simulink model "Version_final_sous_modele"  (R2018b)
settings: Solver=VariableStepAuto  StartTime=0.0  StopTime=10.0  RelTol=1e-3
values from neighbouring files (symbols this model uses):
  fa_clu_pos = [1 1 0.7 0.5 0.3 0 0]    [AxelSplitHEVv4_NEDC_18_06_15.mat]
  fa_clu_pv = [0 0.1 0.3 0.5 0.7 0.9 1]    [AxelSplitHEVv4_NEDC_18_06_15.mat]
  fa_differential_ratio = FDR.fa_differential_ratio    [Algorithme_eff.m]    (also in AxelSplitHEVv4_NEDC_18_06_15.mat = 3.72; fa_differential_ratio.mat = 3.72)
  fa_gearbox_efficiency = 0.92    [AxelSplitHEVv4_NEDC_18_06_15.mat]
  fa_gearbox_ratio = FGR.fa_gearbox_ratio    [Algorithme_eff.m]    (also in AxelSplitHEVv4_NEDC_18_06_15.mat = [0 3.98 2.21 1.47 1.1 0.89 0.75]; fa_gearbox_ratio.mat = [0 3.98 2.21 1.47 1.1 0.89 0.75])
  fa_ice_inertia = 0.058    [AxelSplitHEVv4_NEDC_18_06_15.mat]
  fa_max_tq_clu = 206    [AxelSplitHEVv4_NEDC_18_06_15.mat]
  fa_tau_ice = 0.0333    [AxelSplitHEVv4_NEDC_18_06_15.mat]
  hev_dt = 0.01    [AxelSplitHEVv4_NEDC_18_06_15.mat]
  pla_csat = 1.2    [AxelSplitHEVv4_NEDC_18_06_15.mat]
  pla_equivalent_weight = 1250    [AxelSplitHEVv4_NEDC_18_06_15.mat]
  pla_f = 0.0035272    [AxelSplitHEVv4_NEDC_18_06_15.mat]
  pla_k = 0.0002318    [AxelSplitHEVv4_NEDC_18_06_15.mat]
  pla_kaero = 0.52992    [AxelSplitHEVv4_NEDC_18_06_15.mat]
  pla_max_f_brakes = 1000    [AxelSplitHEVv4_NEDC_18_06_15.mat]
  pla_wheel_radius = 0.314    [AxelSplitHEVv4_NEDC_18_06_15.mat]
  ra_differential_ratio = RDR.ra_differential_ratio    [Algorithme_eff.m]    (also in AxelSplitHEVv4_NEDC_18_06_15.mat = 10; ra_differential_ratio.mat = 10)
  ra_electrical_machine_tau = 0.1    [AxelSplitHEVv4_NEDC_18_06_15.mat]
  ra_transmission_efficiency = 0.92    [AxelSplitHEVv4_NEDC_18_06_15.mat]
undefined symbols (not defined in the file or in its folder): DiscIntNeverNeededParam
libraries: simulink x4
settings Model: Creator=smouline  LastModifiedBy=test
settings SFSimCC: SimUseLocalCustomCode=off
settings RTWCC: RTWUseLocalCustomCode=off
settings CodeAppCC: StateflowObjectComments=on

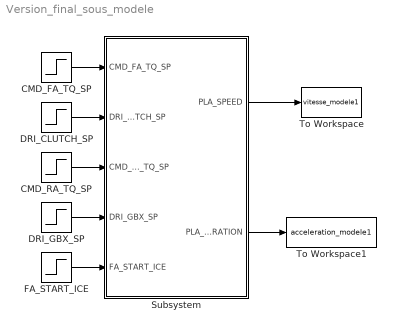
== system Version_final_sous_modele ==
  CMD_FA_TQ_SP : Step  Time=50.1  After=5  SampleTime=0
  CMD_RA_TQ_SP : Step  Time=2  After=10  SampleTime=0
  DRI_CLUTCH_SP : Step  Time=50  Before=1  SampleTime=0
  DRI_GBX_SP : Step  Time=50  Before=1  SampleTime=0
  FA_START_ICE : Step  Time=50  SampleTime=0
  Subsystem : Subsystem
  To Workspace : ToWorkspace  VariableName=vitesse_modele1  SampleTime=-1
  To Workspace1 : ToWorkspace  VariableName=acceleration_modele1  SampleTime=-1
  wires:
  Subsystem/1(PLA_SPEED) -> To Workspace/1
  DRI_GBX_SP/1 -> Subsystem/4(DRI_GBX_SP)
  DRI_CLUTCH_SP/1 -> Subsystem/2(DRI_CLUTCH_SP)
  CMD_FA_TQ_SP/1 -> Subsystem/1(CMD_FA_TQ_SP)
  CMD_RA_TQ_SP/1 -> Subsystem/3(CMD_RA_TQ_SP)
  Subsystem/2(PLA_ACCELERATION) -> To Workspace1/1
  FA_START_ICE/1 -> Subsystem/5(FA_START_ICE)

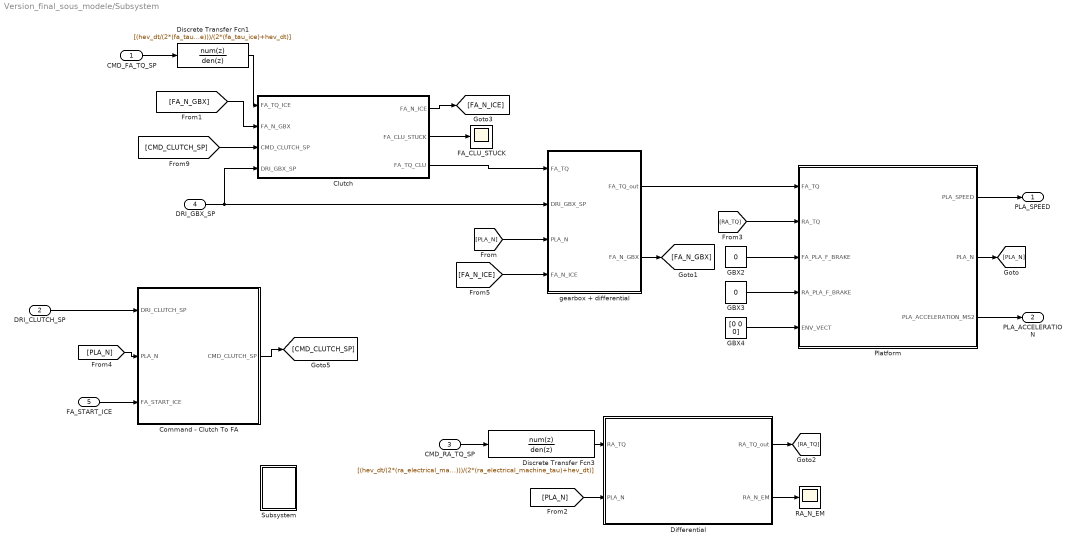
== system Version_final_sous_modele/Subsystem ==
  CMD_FA_TQ_SP : Inport
  DRI_CLUTCH_SP : Inport  Port=2
  CMD_RA_TQ_SP : Inport  Port=3
  DRI_GBX_SP : Inport  Port=4
  FA_START_ICE : Inport  Port=5
  Clutch : Subsystem
  Command - Clutch To FA : Subsystem
  Differential : Subsystem
  Discrete Transfer Fcn1 : DiscreteTransferFcn  Numerator=[(hev_dt/(2*(fa_tau_ice)+hev_dt)) (hev_dt/(2*(fa_tau_ice)+hev_dt))]  Denominator=[1 ((hev_dt-2*(fa_tau_ice)))/(2*(fa_tau_ice)+hev_dt)]  SampleTime=hev_dt
  Discrete Transfer Fcn3 : DiscreteTransferFcn  Numerator=[(hev_dt/(2*(ra_electrical_machine_tau)+hev_dt)) (hev_dt/(2*(ra_electrical_machine_tau)+hev_dt))]  Denominator=[1 ((hev_dt-2*(ra_electrical_machine_tau)))/(2*(ra_electrical_machine_tau)+hev_dt)]  SampleTime=hev_dt
  FA_CLU_STUCK : Scope
  GBX2 : Constant  Value=0
  GBX3 : Constant  Value=0
  GBX4 : Constant  Value=[0 0 0]
  Platform : Subsystem
  RA_N_EM : Scope
  Subsystem : Subsystem
      settings: OpenFcn=open('Documents/Subsystem (extraction of the useful blocs for the clutch’s command).pdf')
      mask Display: fprintf('DOC')
  gearbox + differential : Subsystem
  PLA_SPEED : Outport
  PLA_ACCELERATION : Outport  Port=2
  wires:
  DRI_GBX_SP/1 -> gearbox + differential/2(DRI_GBX_SP), Clutch/4(DRI_GBX_SP)
  Command - Clutch To FA/1("CMD_CLUTCH_SP ") -> [CMD_CLUTCH_SP]
  GBX2/1 -> Platform/3(FA_PLA_F_BRAKE)
  [RA_TQ] -> Platform/2(RA_TQ)
  Differential/2(RA_N_EM) -> RA_N_EM/1
  Platform/3(PLA_ACCELERATION_MS2) -> PLA_ACCELERATION/1
  Differential/1(RA_TQ_out) -> [RA_TQ]
  GBX4/1 -> Platform/5(ENV_VECT)
  gearbox + differential/1("FA_TQ_out ") -> Platform/1(FA_TQ)
  gearbox + differential/2(FA_N_GBX) -> [FA_N_GBX]
  Platform/1(PLA_SPEED) -> PLA_SPEED/1
  [PLA_N] -> gearbox + differential/3(PLA_N)
  [PLA_N] -> Command - Clutch To FA/2(PLA_N)
  Platform/2(PLA_N) -> [PLA_N]
  [FA_N_GBX] -> Clutch/2(FA_N_GBX)
  Discrete Transfer Fcn3/1 -> Differential/1(RA_TQ)
  [FA_N_ICE] -> gearbox + differential/4(FA_N_ICE)
  [PLA_N] -> Differential/2(PLA_N)
  Discrete Transfer Fcn1/1 -> Clutch/1(FA_TQ_ICE)
  Clutch/1(FA_N_ICE) -> [FA_N_ICE]
  CMD_FA_TQ_SP/1 -> Discrete Transfer Fcn1/1
  Clutch/3(FA_TQ_CLU) -> gearbox + differential/1(FA_TQ)
  GBX3/1 -> Platform/4(RA_PLA_F_BRAKE)
  CMD_RA_TQ_SP/1 -> Discrete Transfer Fcn3/1
  [CMD_CLUTCH_SP] -> Clutch/3(CMD_CLUTCH_SP)
  Clutch/2(FA_CLU_STUCK) -> FA_CLU_STUCK/1
  DRI_CLUTCH_SP/1 -> Command - Clutch To FA/1(DRI_CLUTCH_SP)
  FA_START_ICE/1 -> Command - Clutch To FA/3(FA_START_ICE)

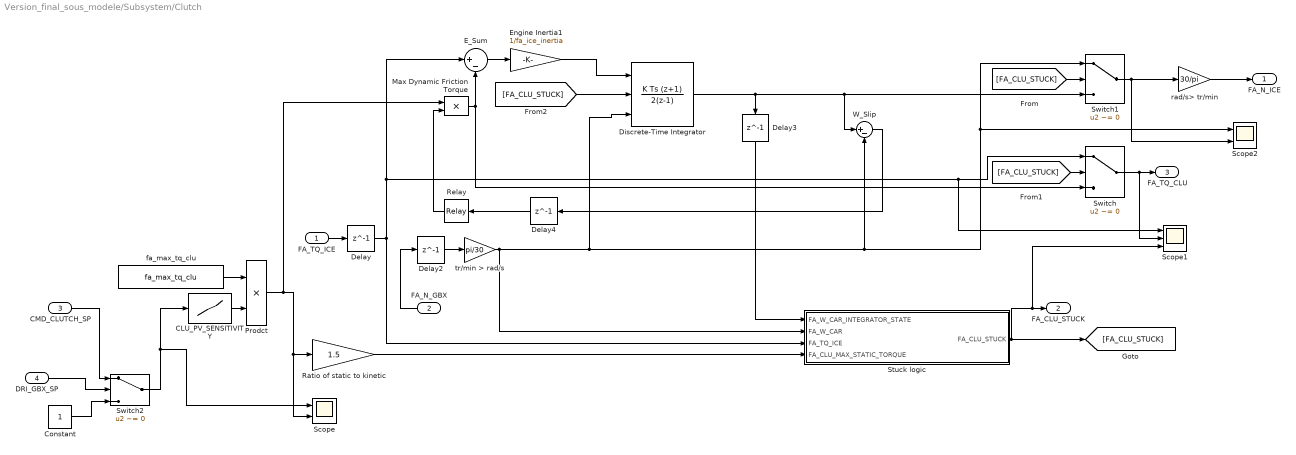
== system Version_final_sous_modele/Subsystem/Clutch ==
  FA_TQ_ICE : Inport
  FA_N_GBX : Inport  Port=2
  CMD_CLUTCH_SP : Inport  Port=3
  DRI_GBX_SP : Inport  Port=4
  " tr/min > rad/s" : Gain  Gain=pi/30  SampleTime=hev_dt
  CLU_PV_SENSITIVITY : Lookup_n-D  NumberOfTableDimensions=1  BreakpointsForDimension1=fa_clu_pv  Table=fa_clu_pos  ExtrapMethod=Clip  UseLastTableValue=on  SampleTime=hev_dt  RndMeth=Simplest  InputSameDT=on
  Constant : Constant
  Delay{,2..4} (4 alike) : Delay  DelayLength=1  SampleTime=hev_dt
  Discrete-Time Integrator : DiscreteIntegrator  IntegratorMethod=Integration: Trapezoidal  ExternalReset=falling  InitialConditionSource=external  SampleTime=hev_dt  ICPrevOutput=DiscIntNeverNeededParam  ICPrevScaledInput=DiscIntNeverNeededParam
  E_Sum : Sum  Inputs=|+-  SampleTime=hev_dt  SaturateOnIntegerOverflow=on  InputSameDT=on  OutDataTypeStr=Inherit: Same as first input
  Engine Inertia1 : Gain  Gain=1/fa_ice_inertia  SampleTime=hev_dt  SaturateOnIntegerOverflow=on  OutDataTypeStr=Inherit: Same as input  ParamDataTypeStr=Inherit: Same as input
  Max Dynamic Friction Torque : Product  SampleTime=hev_dt  SaturateOnIntegerOverflow=on  RndMeth=Zero  InputSameDT=on  OutDataTypeStr=Inherit: Same as first input
  Prodct : Product  SampleTime=hev_dt  RndMeth=Zero
  Ratio of static to kinetic : Gain  Gain=1.5  SampleTime=hev_dt  SaturateOnIntegerOverflow=on  OutDataTypeStr=Inherit: Same as input  ParamDataTypeStr=Inherit: Same as input
  Relay : Relay  OnSwitchValue=0  OffSwitchValue=0  OffOutputValue=-1  SampleTime=hev_dt
  Scope : Scope  NumInputPorts=2
  Scope1 : Scope  NumInputPorts=3
  Scope2 : Scope  NumInputPorts=2
  Stuck logic : Subsystem
  Switch : Switch  Criteria=u2 ~= 0  SampleTime=hev_dt
  Switch1 : Switch  Criteria=u2 ~= 0  SampleTime=hev_dt
  Switch2 : Switch  Criteria=u2 ~= 0
  W_Slip : Sum  Inputs=|+-  SampleTime=hev_dt  SaturateOnIntegerOverflow=on  InputSameDT=on  OutDataTypeStr=Inherit: Same as first input
  fa_max_tq_clu : Constant  Value=fa_max_tq_clu
  rad/s> tr/min : Gain  Gain=30/pi  SampleTime=hev_dt
  FA_N_ICE : Outport
  FA_CLU_STUCK : Outport  Port=2
  FA_TQ_CLU : Outport  Port=3
  wires:
  FA_TQ_ICE/1 -> Delay/1
  Switch1/1 -> Scope2/2, rad/s> tr/min/1
  Switch/1 -> Scope1/2, FA_TQ_CLU/1
  fa_max_tq_clu/1 -> Prodct/1
  Prodct/1 -> Max Dynamic Friction Torque/1, Scope/2, Ratio of static to kinetic/1
  Delay/1 -> E_Sum/1, Scope1/1, Switch/1, Stuck logic/3(FA_TQ_ICE)
  " tr/min > rad/s"/1 -> Discrete-Time Integrator/3, Switch1/1, Scope2/1, W_Slip/2, Stuck logic/2(FA_W_CAR)
  rad/s> tr/min/1 -> FA_N_ICE/1
  Ratio of static to kinetic/1 -> Stuck logic/4(FA_CLU_MAX_STATIC_TORQUE)
  E_Sum/1 -> Engine Inertia1/1
  Engine Inertia1/1 -> Discrete-Time Integrator/1
  Relay/1 -> Max Dynamic Friction Torque/2
  Max Dynamic Friction Torque/1 -> E_Sum/2, Switch/3
  [FA_CLU_STUCK] -> Switch1/2
  [FA_CLU_STUCK] -> Switch/2
  [FA_CLU_STUCK] -> Discrete-Time Integrator/2
  W_Slip/1 -> Delay4/1
  Delay2/1 -> " tr/min > rad/s"/1
  FA_N_GBX/1 -> Delay2/1
  CMD_CLUTCH_SP/1 -> Switch2/1
  Discrete-Time Integrator/1 -> W_Slip/1, Switch1/3, Delay3/1
  Delay3/1 -> Stuck logic/1(FA_W_CAR_INTEGRATOR_STATE)
  Switch2/1 -> Scope/1, CLU_PV_SENSITIVITY/1
  DRI_GBX_SP/1 -> Switch2/2
  Constant/1 -> Switch2/3
  Delay4/1 -> Relay/1
  CLU_PV_SENSITIVITY/1 -> Prodct/2
  Stuck logic/1(FA_CLU_STUCK) -> [FA_CLU_STUCK], Scope1/3, FA_CLU_STUCK/1

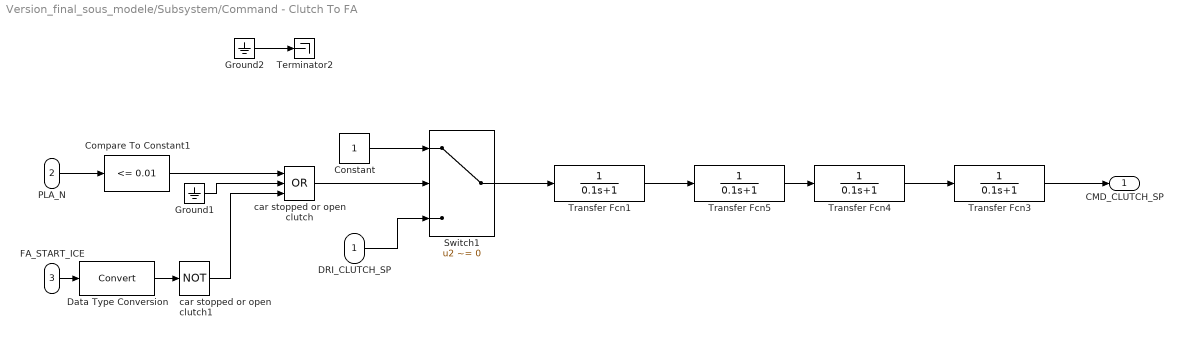
== system Version_final_sous_modele/Subsystem/Command - Clutch To FA ==
  DRI_CLUTCH_SP : Inport
  PLA_N : Inport  Port=2
  FA_START_ICE : Inport  Port=3
  Compare To Constant1 : simulink/Logic and Bit Operations/Compare To Constant  relop=<=  const=0.01  OutDataTypeStr=uint8
  Constant : Constant
  Data Type Conversion : DataTypeConversion
  Ground1 : Ground
  Ground2 : Ground
  Switch1 : Switch  Criteria=u2 ~= 0  Threshold=1
  Terminator2 : Terminator
  Transfer Fcn{1,3..5} (4 alike) : TransferFcn  Denominator=[0.1 1]
  car stopped or open clutch : Logic  Operator=OR  Inputs=3  AllPortsSameDT=off  OutDataTypeStr=boolean
  car stopped or open clutch1 : Logic  Operator=NOT  Inputs=3  AllPortsSameDT=off  OutDataTypeStr=boolean
  "CMD_CLUTCH_SP " : Outport
  wires:
  PLA_N/1 -> Compare To Constant1/1
  FA_START_ICE/1 -> Data Type Conversion/1
  Data Type Conversion/1 -> car stopped or open clutch1/1
  Compare To Constant1/1 -> car stopped or open clutch/1
  Ground1/1 -> car stopped or open clutch/2
  car stopped or open clutch1/1 -> car stopped or open clutch/3
  Ground2/1 -> Terminator2/1
  Constant/1 -> Switch1/1
  car stopped or open clutch/1 -> Switch1/2
  DRI_CLUTCH_SP/1 -> Switch1/3
  Transfer Fcn5/1 -> Transfer Fcn4/1
  Transfer Fcn4/1 -> Transfer Fcn3/1
  Transfer Fcn1/1 -> Transfer Fcn5/1
  Switch1/1 -> Transfer Fcn1/1
  Transfer Fcn3/1 -> "CMD_CLUTCH_SP "/1

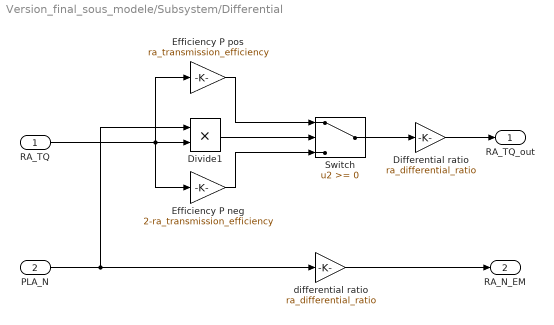
== system Version_final_sous_modele/Subsystem/Differential ==
  RA_TQ : Inport
  PLA_N : Inport  Port=2
  Differential ratio : Gain  Gain=ra_differential_ratio  SampleTime=hev_dt
  Divide1 : Product  SampleTime=hev_dt
  Efficiency P neg : Gain  Gain=2-ra_transmission_efficiency  SampleTime=hev_dt
  Efficiency P pos : Gain  Gain=ra_transmission_efficiency  SampleTime=hev_dt
  Switch : Switch  SampleTime=hev_dt
  differential ratio : Gain  Gain=ra_differential_ratio  SampleTime=hev_dt
  RA_TQ_out : Outport
  RA_N_EM : Outport  Port=2
  wires:
  RA_TQ/1 -> Divide1/2, Efficiency P neg/1, Efficiency P pos/1
  Efficiency P pos/1 -> Switch/1
  Efficiency P neg/1 -> Switch/3
  Divide1/1 -> Switch/2
  Switch/1 -> Differential ratio/1
  PLA_N/1 -> Divide1/1, differential ratio/1
  Differential ratio/1 -> RA_TQ_out/1
  differential ratio/1 -> RA_N_EM/1

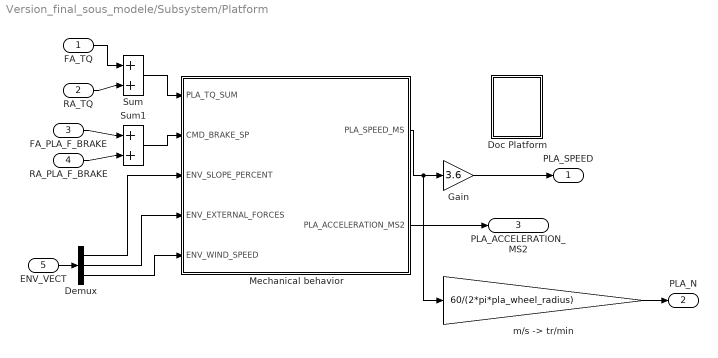
== system Version_final_sous_modele/Subsystem/Platform ==
  FA_TQ : Inport
  RA_TQ : Inport  Port=2
  FA_PLA_F_BRAKE : Inport  Port=3
  RA_PLA_F_BRAKE : Inport  Port=4
  ENV_VECT : Inport  Port=5
  Demux : Demux  Outputs=3
  Doc Platform : Subsystem
      settings: OpenFcn=open('Documents\Platform.pdf')
      mask Display: fprintf('DOC')
  Gain : Gain  Gain=3.6  SampleTime=hev_dt
  Mechanical behavior : Subsystem
  Sum : Sum  Inputs=+|+  SampleTime=hev_dt
  Sum1 : Sum  Inputs=+|+  SampleTime=hev_dt
  "m/s -> tr/min" : Gain  Gain=60/(2*pi*pla_wheel_radius)  SampleTime=hev_dt
  PLA_SPEED : Outport
  PLA_N : Outport  Port=2
  PLA_ACCELERATION_MS2 : Outport  Port=3
  wires:
  Mechanical behavior/1(PLA_SPEED_MS) -> Gain/1, "m/s -> tr/min"/1
  ENV_VECT/1 -> Demux/1
  Gain/1 -> PLA_SPEED/1
  "m/s -> tr/min"/1 -> PLA_N/1
  Sum/1 -> Mechanical behavior/1(PLA_TQ_SUM)
  RA_TQ/1 -> Sum/2
  FA_TQ/1 -> Sum/1
  Sum1/1 -> Mechanical behavior/2(CMD_BRAKE_SP)
  RA_PLA_F_BRAKE/1 -> Sum1/2
  FA_PLA_F_BRAKE/1 -> Sum1/1
  Mechanical behavior/2(PLA_ACCELERATION_MS2) -> PLA_ACCELERATION_MS2/1
  Demux/3 -> Mechanical behavior/5(ENV_WIND_SPEED)
  Demux/2 -> Mechanical behavior/4(ENV_EXTERNAL_FORCES)
  Demux/1 -> Mechanical behavior/3(ENV_SLOPE_PERCENT)

== system Version_final_sous_modele/Subsystem/Subsystem ==

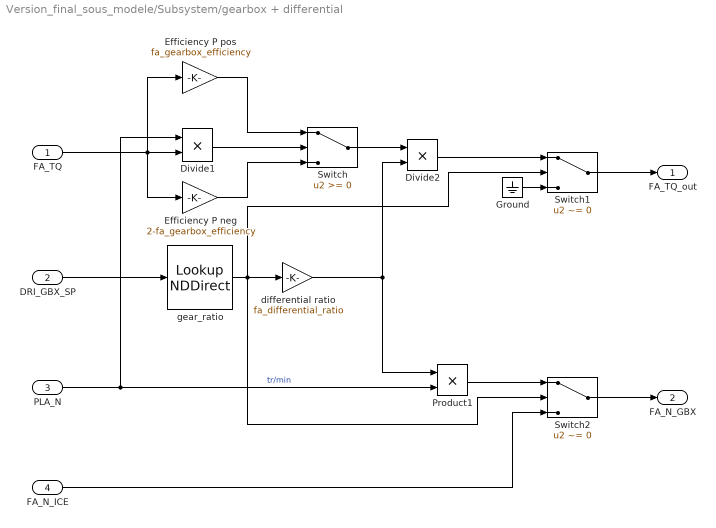
== system Version_final_sous_modele/Subsystem/gearbox + differential ==
  FA_TQ : Inport
  DRI_GBX_SP : Inport  Port=2
  PLA_N : Inport  Port=3
  FA_N_ICE : Inport  Port=4
  " gear_ratio" : LookupNDDirect  NumberOfTableDimensions=1  Table=fa_gearbox_ratio  SampleTime=hev_dt
  Divide1 : Product  SampleTime=hev_dt
  Divide2 : Product  Inputs=**  SampleTime=hev_dt
  Efficiency P neg : Gain  Gain=2-fa_gearbox_efficiency  SampleTime=hev_dt
  Efficiency P pos : Gain  Gain=fa_gearbox_efficiency  SampleTime=hev_dt
  Ground : Ground
  Product1 : Product  SampleTime=hev_dt  RndMeth=Zero
  Switch : Switch  SampleTime=hev_dt
  Switch1 : Switch  Criteria=u2 ~= 0  SampleTime=hev_dt
  Switch2 : Switch  Criteria=u2 ~= 0  SampleTime=hev_dt
  differential ratio : Gain  Gain=fa_differential_ratio  SampleTime=hev_dt
  "FA_TQ_out " : Outport
  FA_N_GBX : Outport  Port=2
  wires:
  DRI_GBX_SP/1 -> " gear_ratio"/1
  " gear_ratio"/1 -> Switch1/2, differential ratio/1, Switch2/2
  differential ratio/1 -> Divide2/2, Product1/1
  Divide2/1 -> Switch1/1
  FA_TQ/1 -> Divide1/2, Efficiency P neg/1, Efficiency P pos/1
  Efficiency P pos/1 -> Switch/1
  Efficiency P neg/1 -> Switch/3
  Divide1/1 -> Switch/2
  Switch/1 -> Divide2/1
  Product1/1 -> Switch2/1
  PLA_N/1 -> Product1/2, Divide1/1  "tr/min"
  Switch1/1 -> "FA_TQ_out "/1
  Ground/1 -> Switch1/3
  Switch2/1 -> FA_N_GBX/1
  FA_N_ICE/1 -> Switch2/3

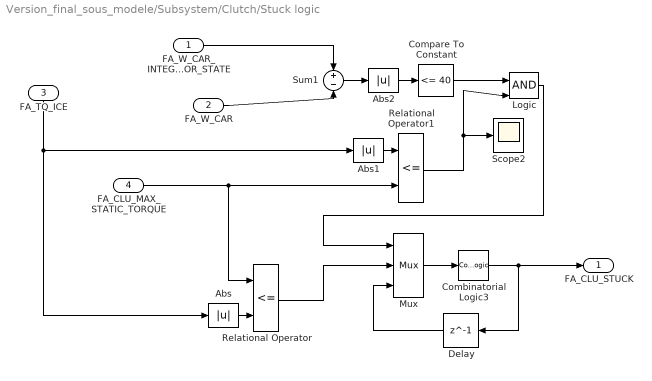
== system Version_final_sous_modele/Subsystem/Clutch/Stuck logic ==
  FA_W_CAR_INTEGRATOR_STATE : Inport
  FA_W_CAR : Inport  Port=2
  FA_TQ_ICE : Inport  Port=3
  FA_CLU_MAX_STATIC_TORQUE : Inport  Port=4
  Abs : Abs  SampleTime=hev_dt  SaturateOnIntegerOverflow=on
  Abs1 : Abs  SampleTime=hev_dt  SaturateOnIntegerOverflow=on
  Abs2 : Abs  SampleTime=hev_dt  SaturateOnIntegerOverflow=on
  Combinatorial Logic3 : CombinatorialLogic  Description=TRUTH_TABLE_FROM_FABIEN  TruthTable=[0;1;0;0;1;1;0;1]  SampleTime=hev_dt
  Compare To Constant : simulink/Logic and Bit Operations/Compare To Constant  relop=<=  const=40  OutDataTypeStr=boolean
  Delay : Delay  DelayLength=1  SampleTime=hev_dt
  Logic : Logic  IconShape=distinctive  SampleTime=hev_dt
  Mux : Mux  Inputs=3
  Relational Operator : RelationalOperator  Operator=<=  SampleTime=hev_dt  RndMeth=Nearest  InputSameDT=on
  Relational Operator1 : RelationalOperator  Operator=<=  SampleTime=hev_dt  RndMeth=Nearest  InputSameDT=on
  Scope2 : Scope
  Sum1 : Sum  Inputs=+-  SampleTime=hev_dt  SaturateOnIntegerOverflow=on  InputSameDT=on  OutDataTypeStr=Inherit: Same as first input
  FA_CLU_STUCK : Outport
  wires:
  FA_CLU_MAX_STATIC_TORQUE/1 -> Relational Operator1/2, Relational Operator/1
  Sum1/1 -> Abs2/1
  Abs1/1 -> Relational Operator1/1
  Delay/1 -> Mux/3
  Combinatorial Logic3/1 -> Delay/1, FA_CLU_STUCK/1
  Mux/1 -> Combinatorial Logic3/1
  Abs/1 -> Relational Operator/2
  Relational Operator/1 -> Mux/2
  Logic/1 -> Mux/1
  Abs2/1 -> Compare To Constant/1
  Compare To Constant/1 -> Logic/1
  Relational Operator1/1 -> Scope2/1, Logic/2
  FA_TQ_ICE/1 -> Abs1/1, Abs/1
  FA_W_CAR_INTEGRATOR_STATE/1 -> Sum1/1
  FA_W_CAR/1 -> Sum1/2

== system Version_final_sous_modele/Subsystem/Platform/Doc Platform ==

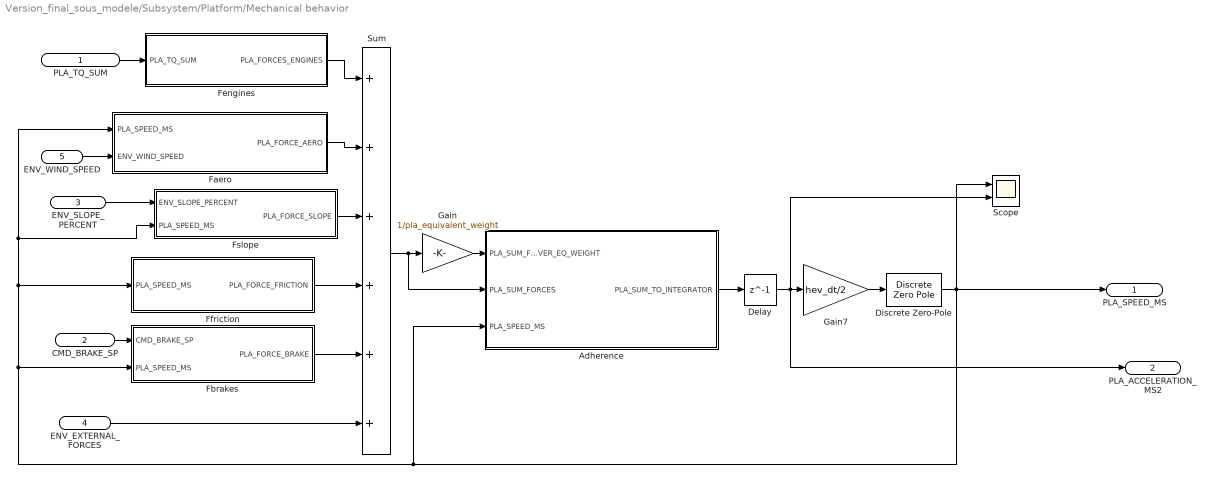
== system Version_final_sous_modele/Subsystem/Platform/Mechanical behavior ==
  PLA_TQ_SUM : Inport  Tag=tag
  CMD_BRAKE_SP : Inport  Port=2
  ENV_SLOPE_PERCENT : Inport  Port=3
  ENV_EXTERNAL_FORCES : Inport  Port=4
  ENV_WIND_SPEED : Inport  Port=5
  Adherence : Subsystem
  Delay : Delay  DelayLength=1  SampleTime=hev_dt
  Discrete Zero-Pole : DiscreteZeroPole  Zeros=[-1]  Poles=[1]  Gain=1  SampleTime=hev_dt
  Faero : Subsystem
  Fbrakes : Subsystem
  Fengines : Subsystem
  Ffriction : Subsystem
  Fslope : Subsystem
  Gain : Gain  Gain=1/pla_equivalent_weight  SampleTime=hev_dt
  Gain7 : Gain  Gain=hev_dt/2  SampleTime=hev_dt
  Scope : Scope  NumInputPorts=2
  Sum : Sum  Inputs=++++++  SampleTime=hev_dt
  PLA_SPEED_MS : Outport
  PLA_ACCELERATION_MS2 : Outport  Port=2
  wires:
  Gain/1 -> Adherence/1(PLA_SUM_FORCES_OVER_EQ_WEIGHT)
  Ffriction/1(PLA_FORCE_FRICTION) -> Sum/4
  Sum/1 -> Gain/1, Adherence/2(PLA_SUM_FORCES)
  Discrete Zero-Pole/1 -> Scope/1, Adherence/3(PLA_SPEED_MS), Fbrakes/2(PLA_SPEED_MS), Ffriction/1(PLA_SPEED_MS), Faero/1(PLA_SPEED_MS), Fslope/2(PLA_SPEED_MS), PLA_SPEED_MS/1
  ENV_SLOPE_PERCENT/1 -> Fslope/1(ENV_SLOPE_PERCENT)
  ENV_WIND_SPEED/1 -> Faero/2(ENV_WIND_SPEED)
  PLA_TQ_SUM/1 -> Fengines/1(PLA_TQ_SUM)
  Fengines/1(PLA_FORCES_ENGINES) -> Sum/1
  Faero/1(PLA_FORCE_AERO) -> Sum/2
  Fslope/1(PLA_FORCE_SLOPE) -> Sum/3
  ENV_EXTERNAL_FORCES/1 -> Sum/6
  CMD_BRAKE_SP/1 -> Fbrakes/1(CMD_BRAKE_SP)
  Fbrakes/1(PLA_FORCE_BRAKE) -> Sum/5
  Adherence/1(PLA_SUM_TO_INTEGRATOR) -> Delay/1
  Delay/1 -> Scope/2, PLA_ACCELERATION_MS2/1, Gain7/1
  Gain7/1 -> Discrete Zero-Pole/1

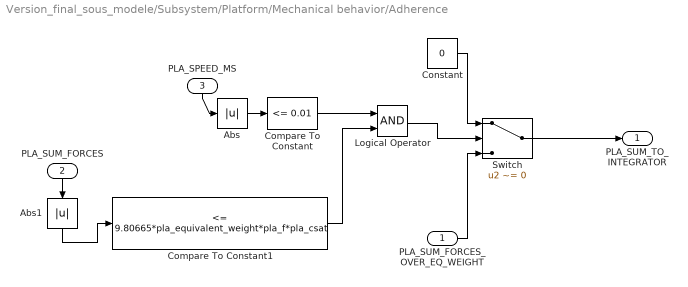
== system Version_final_sous_modele/Subsystem/Platform/Mechanical behavior/Adherence ==
  PLA_SUM_FORCES_OVER_EQ_WEIGHT : Inport
  PLA_SUM_FORCES : Inport  Port=2
  PLA_SPEED_MS : Inport  Port=3
  Abs : Abs  SampleTime=hev_dt
  Abs1 : Abs  SampleTime=hev_dt
  Compare To Constant : simulink/Logic and Bit Operations/Compare To Constant  relop=<=  const=0.01  OutDataTypeStr=uint8
  Compare To Constant1 : simulink/Logic and Bit Operations/Compare To Constant  relop=<=  const=9.80665*pla_equivalent_weight*pla_f*pla_csat  OutDataTypeStr=uint8
  Constant : Constant  Value=0
  Logical Operator : Logic  AllPortsSameDT=off  OutDataTypeStr=boolean  SampleTime=hev_dt
  Switch : Switch  Criteria=u2 ~= 0  SampleTime=hev_dt
  PLA_SUM_TO_INTEGRATOR : Outport
  wires:
  PLA_SUM_FORCES_OVER_EQ_WEIGHT/1 -> Switch/3
  Switch/1 -> PLA_SUM_TO_INTEGRATOR/1
  PLA_SPEED_MS/1 -> Abs/1
  PLA_SUM_FORCES/1 -> Abs1/1
  Abs1/1 -> Compare To Constant1/1
  Abs/1 -> Compare To Constant/1
  Constant/1 -> Switch/1
  Compare To Constant1/1 -> Logical Operator/2
  Logical Operator/1 -> Switch/2
  Compare To Constant/1 -> Logical Operator/1

== system Version_final_sous_modele/Subsystem/Platform/Mechanical behavior/Faero ==
  PLA_SPEED_MS : Inport
  ENV_WIND_SPEED : Inport  Port=2
  Gain : Gain  Gain=-1  SampleTime=hev_dt
  Gain1 : Gain  Gain=pla_kaero  SampleTime=hev_dt
  Product : Product  SampleTime=hev_dt
  Product1 : Product  SampleTime=hev_dt
  Sign : Signum  SampleTime=hev_dt
  Sum : Sum  Inputs=+|+  SampleTime=hev_dt
  PLA_FORCE_AERO : Outport
  wires:
  PLA_SPEED_MS/1 -> Sign/1, Sum/1
  ENV_WIND_SPEED/1 -> Sum/2
  Sum/1 -> Product/2, Product/1
  Product/1 -> Gain1/1
  Gain1/1 -> Product1/2
  Product1/1 -> Gain/1
  Sign/1 -> Product1/1
  Gain/1 -> PLA_FORCE_AERO/1

== system Version_final_sous_modele/Subsystem/Platform/Mechanical behavior/Fbrakes ==
  CMD_BRAKE_SP : Inport
  PLA_SPEED_MS : Inport  Port=2
  Gain2 : Gain  Gain=-1  SampleTime=hev_dt
  Product1 : Product  SampleTime=hev_dt
  Saturation : Saturate  UpperLimit=pla_max_f_brakes  LowerLimit=0
  Sign : Signum  SampleTime=hev_dt
  PLA_FORCE_BRAKE : Outport
  wires:
  CMD_BRAKE_SP/1 -> Saturation/1
  PLA_SPEED_MS/1 -> Sign/1
  Sign/1 -> Product1/1
  Product1/1 -> Gain2/1
  Gain2/1 -> PLA_FORCE_BRAKE/1
  Saturation/1 -> Product1/2

== system Version_final_sous_modele/Subsystem/Platform/Mechanical behavior/Fengines ==
  PLA_TQ_SUM : Inport
  Gain1 : Gain  Gain=1/pla_wheel_radius  SampleTime=hev_dt
  PLA_FORCES_ENGINES : Outport
  wires:
  PLA_TQ_SUM/1 -> Gain1/1
  Gain1/1 -> PLA_FORCES_ENGINES/1

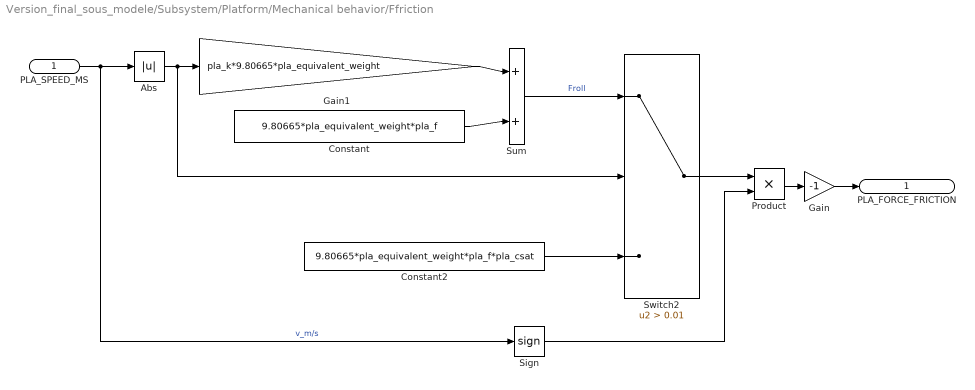
== system Version_final_sous_modele/Subsystem/Platform/Mechanical behavior/Ffriction ==
  PLA_SPEED_MS : Inport
  Abs : Abs  SampleTime=hev_dt
  Constant : Constant  Value=9.80665*pla_equivalent_weight*pla_f
  Constant2 : Constant  Value=9.80665*pla_equivalent_weight*pla_f*pla_csat
  Gain : Gain  Gain=-1  SampleTime=hev_dt
  Gain1 : Gain  Gain=pla_k*9.80665*pla_equivalent_weight  SampleTime=hev_dt
  Product : Product  SampleTime=hev_dt
  Sign : Signum  SampleTime=hev_dt
  Sum : Sum  Inputs=+|+  SampleTime=hev_dt
  Switch2 : Switch  Criteria=u2 > Threshold  Threshold=0.01  SampleTime=hev_dt
  PLA_FORCE_FRICTION : Outport
  wires:
  PLA_SPEED_MS/1 -> Abs/1, Sign/1  "v_m/s"
  Gain1/1 -> Sum/1
  Constant/1 -> Sum/2
  Abs/1 -> Gain1/1, Switch2/2
  Switch2/1 -> Product/1
  Product/1 -> Gain/1
  Sign/1 -> Product/2
  Gain/1 -> PLA_FORCE_FRICTION/1
  Sum/1 -> Switch2/1  "Froll"
  Constant2/1 -> Switch2/3

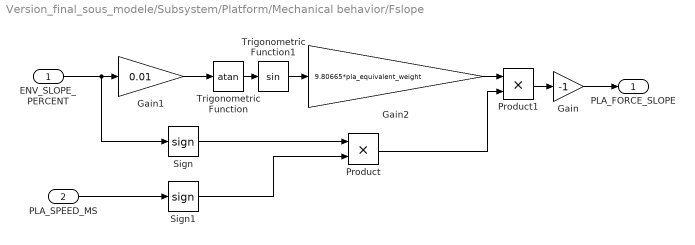
== system Version_final_sous_modele/Subsystem/Platform/Mechanical behavior/Fslope ==
  ENV_SLOPE_PERCENT : Inport
  PLA_SPEED_MS : Inport  Port=2
  Gain : Gain  Gain=-1  SampleTime=hev_dt
  Gain1 : Gain  Gain=0.01  SampleTime=hev_dt
  Gain2 : Gain  Gain=9.80665*pla_equivalent_weight  SampleTime=hev_dt
  Product : Product  SampleTime=hev_dt
  Product1 : Product  SampleTime=hev_dt
  Sign : Signum  SampleTime=hev_dt
  Sign1 : Signum  SampleTime=hev_dt
  Trigonometric Function : Trigonometry  Operator=atan  SampleTime=hev_dt
  Trigonometric Function1 : Trigonometry  SampleTime=hev_dt
  PLA_FORCE_SLOPE : Outport
  wires:
  ENV_SLOPE_PERCENT/1 -> Sign/1, Gain1/1
  Gain1/1 -> Trigonometric Function/1
  Trigonometric Function/1 -> Trigonometric Function1/1
  Trigonometric Function1/1 -> Gain2/1
  Gain/1 -> PLA_FORCE_SLOPE/1
  PLA_SPEED_MS/1 -> Sign1/1
  Sign/1 -> Product/1
  Sign1/1 -> Product/2
  Gain2/1 -> Product1/1
  Product/1 -> Product1/2
  Product1/1 -> Gain/1
